simulink model "A8_KGT_Stellantrieb"  (R2017b)
settings: Solver=ode45  StartTime=0.0  StopTime=5  MaxStep=1e-3  RelTol=1e-3  EnableMultiTasking=on
values from neighbouring files (symbols this model uses):
  CD = 1e1    (= 10)    [A14_Konstanten.m]    (also in A17_Konstanten.m = 100; A8_Konstanten.m = 20; A9_Konstanten.m = 0.1)
  CF = 1e4    (= 10000)    [A13_Konstanten.m]    (also in A14_Konstanten.m; A17_Konstanten.m = 50000; A8_Konstanten.m = 10000000; A9_Konstanten.m)
  D = CD/(2*sqrt(CF*m1))    [A8_Konstanten.m]
  K = P*CD/(2*pi*m1)    (= 0.00318309886184)    [A8_Konstanten.m]
  m1 = 1    [A13_Konstanten.m]    (also in A14_Konstanten.m; A17_Konstanten.m = 4; A8_Konstanten.m = 20)
  P = 0.02    [A8_Konstanten.m]    (also in A9_Konstanten.m = 0.04)
  p1 = -D*w0 + j*w0*sqrt(1-D^2)    [A8_Konstanten.m]
  p2 = -D*w0 - j*w0*sqrt(1-D^2)    [A8_Konstanten.m]
  q1 = -CF/CD    (= -500000)    [A8_Konstanten.m]
  w0 = sqrt(CF/m1)    [A8_Konstanten.m]
undefined symbols (not defined in the file or in its folder): sigbuilder_block
settings Model: Creator=jbaur  LastModifiedBy=jbaur
settings DataIOCC: ExternalInput=X1  SaveFormat=StructureWithTime  InspectSignalLogs=on  SignalLoggingName=sigsOut
settings OptimizationCC: ExpressionDepthLimit=2147483647  InitFltsAndDblsToZero=on  LifeSpan=inf
settings DebuggingCC: SaveWithParameterizedLinksMsg=none  SignalResolutionControl=TryResolveAllWithWarning  MultiTaskDSMMsg=warning  MultiTaskCondExecSysMsg=none  StateNameClashWarn=warning  SFUnexpectedBacktrackingDiag=warning  SFNoUnconditionalDefaultTransitionDiag=warning  SFExecutionAtInitializationDiag=none
settings HardwareCC: ProdBitPerPointer=32  ProdBitPerSizeT=32  ProdBitPerPtrDiffT=32  ProdLargestAtomicFloat=None  ProdIntDivRoundTo=Undefined  ProdEndianess=Unspecified  ProdWordSize=32  ProdHWDeviceType=32-bit Generic  TargetUnknown=on
settings ModelReferenceCC: PropagateSignalLabelsOutOfModel=off
settings CodeAppCC: StateflowObjectComments=on
settings GRTTargetCC: TargetFcnLib=ansi_tfl_tmw.mat  TargetLangStandard=C89/C90 (ANSI)  ModelReferenceCompliant=off  GeneratePreprocessorConditionals=Disable all  CombineOutputUpdateFcns=off  MatFileLogging=off  GRTInterface=on
settings ConfigComp: CovMetricSettings=dw  CovHtmlReporting=on  CovSaveCumulativeToWorkspaceVar=on  CovSaveSingleToWorkspaceVar=on  CovExternalEMLEnable=off  CovSFcnEnable=off

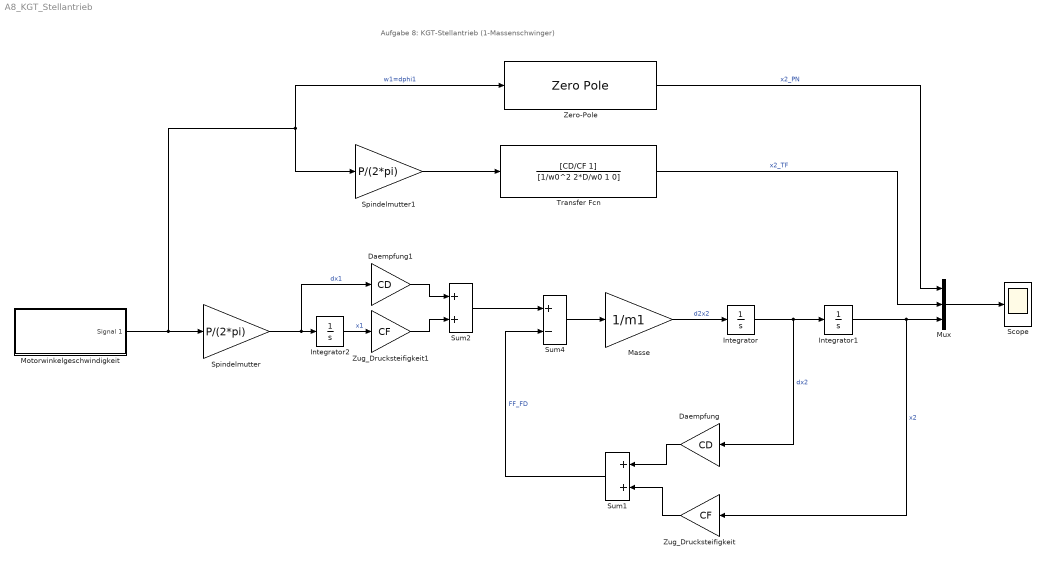
== system A8_KGT_Stellantrieb ==
  note: Aufgabe 8: KGT-Stellantrieb (1-Massenschwinger)
  Daempfung : Gain  Gain=CD
  Daempfung1 : Gain  Gain=CD
  Integrator : Integrator
  Integrator1 : Integrator
  Integrator2 : Integrator
  Masse : Gain  Gain=1/m1
  Motorwinkelgeschwindigkeit : Subsystem  Tag=STV Subsys  LoadFcn=sigbuilder_block('load');  StartFcn=sigbuilder_block('start');  StopFcn=sigbuilder_block('stop');  ClipboardFcn=sigbuilder_block('clipboard');  mask(Sigbuilder block){tuvar=[0:10]}
      mask help: Sigbuilder GUI
      mask init:
      | if ~strcmp(get_param(bdroot(gcbh),'SimulationStatus'),'stopped') tuvar = sigbuilder_block('maskInit'); end
      settings: CopyFcn=sigbuilder_block('copy');  DeleteFcn=sigbuilder_block('delete');  ModelCloseFcn=sigbuilder_block('modelClose');  PreSaveFcn=sigbuilder_block('preSave');  PauseFcn=sigbuilder_block('pause')  ContinueFcn=sigbuilder_block('continue')  NameChangeFcn=sigbuilder_block('namechange');  OpenFcn=sigbuilder_block('open',[49.5 50.25 519.75 399.75 ]);  CloseFcn=sigbuilder_block('close');
      mask Display: plot(0, 0, 100, 100,[2, 2, 32, 32, 2], [68, 8, 8, 68, 68],[32, 2], [38, 38], [32, 19, 2],[53, 60, 44], [32, 17, 17, 2],[16, 16, 31, 31]);txt = getActiveGroup(gcbh);text(2, 100, txt,'verticalAlignment', 'top');
  Mux : Mux  Inputs=3
  Scope : Scope
  Spindelmutter : Gain  Gain=P/(2*pi)
  Spindelmutter1 : Gain  Gain=P/(2*pi)
  Sum1 : Sum
  Sum2 : Sum
  Sum4 : Sum  Inputs=+-
  Transfer Fcn : TransferFcn  Numerator=[CD/CF 1]  Denominator=[1/w0^2 2*D/w0 1 0]
  Zero-Pole : ZeroPole  Zeros=[q1]  Poles=[p1 p2 0]  Gain=[K]
  Zug_Drucksteifigkeit : Gain  Gain=CF
  Zug_Drucksteifigkeit1 : Gain  Gain=CF
  wires:
  Masse/1 -> Integrator/1  "d2x2"
  Integrator/1 -> Daempfung/1, Integrator1/1  "dx2"
  Integrator1/1 -> Mux/3, Zug_Drucksteifigkeit/1  "x2"
  Sum4/1 -> Masse/1
  Zug_Drucksteifigkeit/1 -> Sum1/2
  Daempfung/1 -> Sum1/1
  Spindelmutter/1 -> Daempfung1/1, Integrator2/1  "dx1"
  Motorwinkelgeschwindigkeit/1(Signal 1) -> Zero-Pole/1, Spindelmutter1/1, Spindelmutter/1  "w1=dphi1"
  Sum1/1 -> Sum4/2  "FF_FD"
  Integrator2/1 -> Zug_Drucksteifigkeit1/1  "x1"
  Sum2/1 -> Sum4/1
  Zug_Drucksteifigkeit1/1 -> Sum2/2
  Daempfung1/1 -> Sum2/1
  Mux/1 -> Scope/1
  Transfer Fcn/1 -> Mux/2  "x2_TF"
  Zero-Pole/1 -> Mux/1  "x2_PN"
  Spindelmutter1/1 -> Transfer Fcn/1

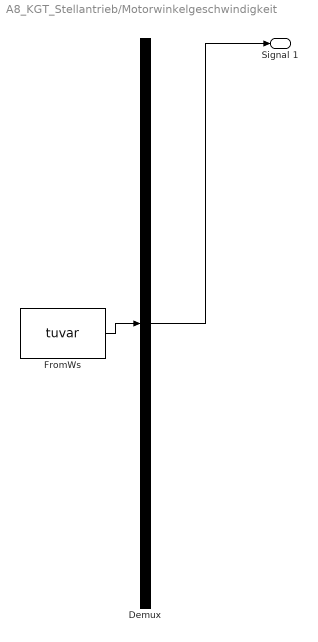
== system A8_KGT_Stellantrieb/Motorwinkelgeschwindigkeit ==
  Demux : Demux  Tag=STV Demux  Outputs=1
  FromWs : FromWorkspace  Tag=STV FromWs  VariableName=tuvar  SampleTime=0
      SigBuilderData=|
      | dataSet.timeRange = [0 4]
      | dataSet.name = 'Group 1'
      | sbobj.Groups.Name = 'Group 1'
      | sbobj.Groups.Signals.Name = 'Signal 1'
      | sbobj.Groups.Signals.XData = [0 1 2 3 4]
      | sbobj.Groups.Signals.YData = [0 62.8318530718 62.8318530718 0 0]
      | sbobj.Groups.TimeRange = [0 4]
  Signal 1 : Outport  Tag=STV Outport
  wires:
  Demux/1 -> Signal 1/1
  FromWs/1 -> Demux/1
